simulink model "BMS_State_AutoBuild"  (R2026a)
settings: Solver=VariableStepAuto
settings Model: Creator=tastytaco  LastModifiedBy=tastytaco

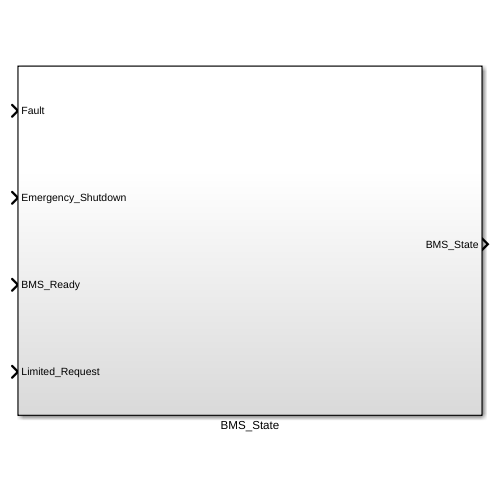
[thumbnail: Simulink's stored preview of the top-level diagram]
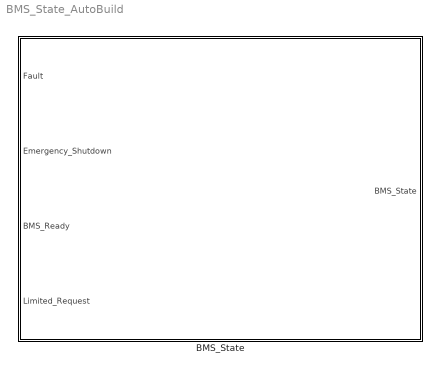
== system BMS_State_AutoBuild ==
  BMS_State : Subsystem

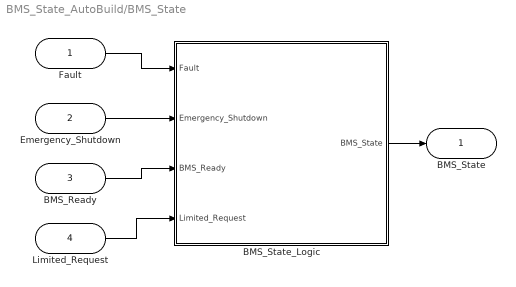
== system BMS_State_AutoBuild/BMS_State ==
  Fault : Inport
  Emergency_Shutdown : Inport  Port=2
  BMS_Ready : Inport  Port=3
  Limited_Request : Inport  Port=4
  BMS_State_Logic : MATLAB Function  TreatAsAtomicUnit=on
  BMS_State : Outport
  wires:
  BMS_State_Logic/1(BMS_State) -> BMS_State/1
  BMS_Ready/1 -> BMS_State_Logic/3(BMS_Ready)
  Limited_Request/1 -> BMS_State_Logic/4(Limited_Request)
  Emergency_Shutdown/1 -> BMS_State_Logic/2(Emergency_Shutdown)
  Fault/1 -> BMS_State_Logic/1(Fault)

== matlab function BMS_State_AutoBuild/BMS_State/BMS_State_Logic ==
  data: Fault input; BMS_State output; Emergency_Shutdown input; BMS_Ready input; Limited_Request input
function BMS_State = fcn(Fault, Emergency_Shutdown, BMS_Ready, Limited_Request)

% BMS State Codes
% 0 = INIT
% 1 = NORMAL
% 2 = LIMITED
% 3 = FAULT
% 4 = SHUTDOWN

% Highest priority state is SHUTDOWN.
if Emergency_Shutdown
    BMS_State = 4;

% Protection fault.
elseif Fault
    BMS_State = 3;

% BMS has not completed its ready condition.
elseif ~BMS_Ready
    BMS_State = 0;

% BMS is operating but under a limitation.
elseif Limited_Request
    BMS_State = 2;

% Normal operation.
else
    BMS_State = 1;
end

end
